simulink model "CobiCalibration"  (R2020b)
settings: Solver=FixedStepDiscrete  StartTime=0.0  StopTime=inf  FixedStep=0.01  RelTol=1e-3  EnableMultiTasking=on
libraries: simulink x9
settings Model: DataDictionary=CobiCalibrationDD.sldd  EnableAccessToBaseWorkspace=off  DataTypeOverride=Off  DataTypeOverrideAppliesTo=Floating-point  MinMaxOverflowLogging=ForceOff  Creator=stj1si  LastModifiedBy=snj7rt
settings DataIOCC: SaveFormat=Array  SaveOutput=off  SignalLogging=off  SaveTime=off  ReturnWorkspaceOutputs=off
settings OptimizationCC: DefaultParameterBehavior=Inlined  DefaultUnderspecifiedDataType=single  InlineInvariantSignals=on  EnhancedBackFolding=on  CachingGlobalReferences=on  ExpressionDepthLimit=2147483647  NoFixptDivByZeroProtection=on  EfficientFloat2IntCast=on  LifeSpan=1  SimCompilerOptimization=on  EfficientTunableParamExpr=on
settings DebuggingCC: SolverPrmCheckMsg=warning  ParameterPrecisionLossMsg=none  AllowSymbolicDim=off  StateNameClashWarn=warning  SFUnexpectedBacktrackingDiag=warning  SFNoUnconditionalDefaultTransitionDiag=warning  SFExecutionAtInitializationDiag=none  ArithmeticOperatorsInVariantConditions=warning
settings HardwareCC: ProdBitPerPointer=32  ProdBitPerSizeT=32  ProdBitPerPtrDiffT=32  ProdLargestAtomicInteger=Long  ProdLargestAtomicFloat=Double  ProdEndianess=BigEndian  ProdWordSize=32  ProdHWDeviceType=Freescale->32-bit PowerPC
settings ModelReferenceCC: ModelReferenceNumInstancesAllowed=Single  PropagateSignalLabelsOutOfModel=off
settings SFSimCC: SimUseLocalCustomCode=off  MATLABDynamicMemAlloc=off  CustomCodeUndefinedFunction=UseInterfaceOnly
settings RTWCC: Description=Embedded Coder  SystemTargetFile=ert.tlc  GenCodeOnly=on  TemplateMakefile=ert_default_tmf  GenerateReport=on  RTWUseLocalCustomCode=off  IncludeHyperlinkInReport=on  LaunchReport=on  GenerateTraceInfo=on  GenerateTraceReport=on  GenerateTraceReportSl=on  GenerateTraceReportSf=on  GenerateTraceReportEml=on
settings CodeAppCC: IgnoreCustomStorageClasses=off  CustomSymbolStrType=$N$R$M  CustomSymbolStrFcnArg=COCA_rt$I$N$M  CustomSymbolStrBlkIO=COCA_rtb_$N$M  StateflowObjectComments=on  InternalIdentifier=Classic
settings ERTTargetCC: TargetLangStandard=C99 (ISO)  MultiwordLength=2048  GenerateSampleERTMain=on  IncludeMdlTerminateFcn=off  CombineSignalStateStructs=on  SuppressErrorStatus=on  SupportNonFinite=off  SupportComplex=off  CastingMode=Standards  InlinedParameterPlacement=NonHierarchical  ERTSrcFileBannerTemplate=ert_code_template_ebike.cgt  ERTCustomFileTemplate=example_file_process.tlc  ERTFilePackagingFormat=Compact  PreserveExternInFcnDecls=off  SuppressUnreachableDefaultCases=off  EnableSignedLeftShifts=off  EnableSignedRightShifts=off  IndentStyle=Allman  EnableUserReplacementTypes=on
settings ConfigComp: CovEnable=on  CovScope=ReferencedModels  CovIncludeTopModel=off  CovMetricSettings=dw  CovHTMLOptions=-sRT=1 -sVT=0 -aTS=1 -bRG=1 -bTC=1 -hTR=0 -nFC=0 -nFD=1 -scm=1 -bcm=1 -xEv=0 -xEM=0  CovSaveCumulativeToWorkspaceVar=on  CovSaveSingleToWorkspaceVar=on  CovModelRefEnable=all  CovSFcnEnable=off

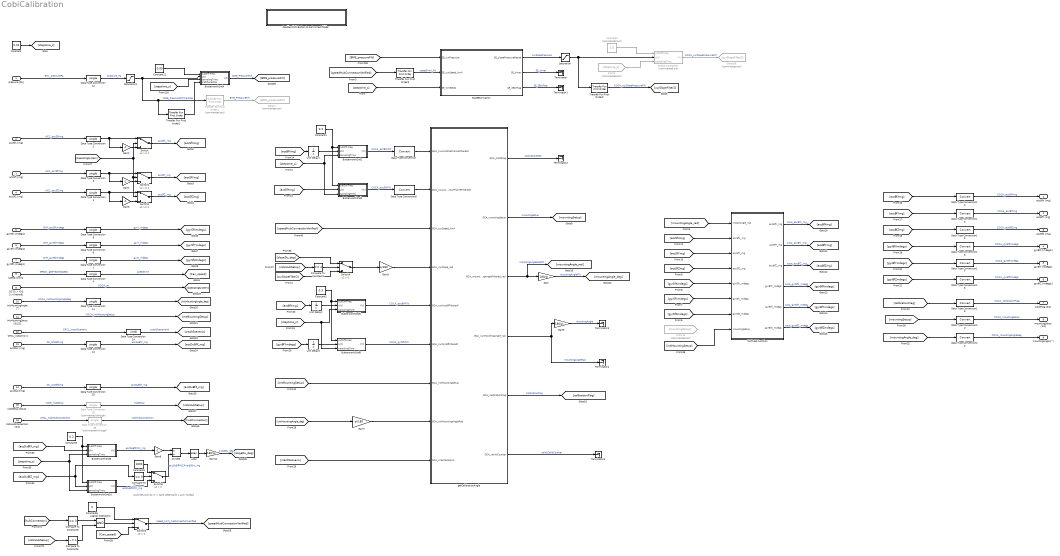
== system CobiCalibration ==
  note: avoid devision by 0 -> take 1000mg for z axis instead
  "pressure [Pa] " : Inport
  accSfX [mg] : Inport  Port=2
  accSfY [mg] : Inport  Port=3
  accSfZ [mg] : Inport  Port=4
  gyrSfX [mdeg/s] : Inport  Port=5
  gyrSfY [mdeg/s] : Inport  Port=6
  gyrSfZ [mdeg/s] : Inport  Port=7
  speed [km/h] : Inport  Port=8
  "OS [1-> iOS, 2->Android]" : Inport  Port=9
  initMountingAngle [°] : Inport  Port=10
  initMountingSetup [0/1/2] : Inport  Port=11
  " CRCL_sceanrio []" : Inport  Port=12
  accDuX [mg] : Inport  Port=13
  accDuZ [mg] : Inport  Port=14
  cobiSetup [0/1/2] : Inport  Port=15
  CobiHubConnection [0/1] : Inport  Port=16
  Atan : Trigonometry  Operator=atan
  Butterworth2nd1 : Subsystem
  Butterworth2nd10 : Subsystem
  Butterworth2nd2 : Subsystem
  Butterworth2nd4 : Subsystem
  Butterworth2nd5 : Subsystem
  Butterworth2nd7 : Subsystem  Commented=on
  Butterworth2nd8 : Subsystem
  Butterworth2nd9 : Subsystem
  Compare To Constant : simulink/Logic and Bit Operations/Compare To Constant  relop===  const=0  OutDataTypeStr=boolean
  Compare To Constant1 : simulink/Logic and Bit Operations/Compare To Constant  relop===  const=2  OutDataTypeStr=boolean
  Compare To Constant6 : simulink/Logic and Bit Operations/Compare To Constant  relop===  const=0  OutDataTypeStr=boolean
  Compare To Constant8 : simulink/Logic and Bit Operations/Compare To Constant  relop=~=  const=1  OutDataTypeStr=boolean
  Constant : Constant  Value=0.01
  Constant1 : Constant  Value=0.3
  Constant11 : Constant  Value=0.05
  Constant2 : Constant  Value=0.3
  Constant3 : Constant  Value=0.2
  Constant4 : Constant  Commented=on  Value=0.5
  Constant5 : Constant  Value=0  OutDataTypeStr=single
  Constant6 : Constant  Value=1000
  Data Type Conversion{,5,10,13,15..19,22..23} (11 alike) : DataTypeConversion  RndMeth=Zero
  Data Type Conversion{1..4,7..9,11..12,24..25} (11 alike) : DataTypeConversion  OutDataTypeStr=single
  Data Type Conversion14 : DataTypeConversion  OutDataTypeStr=uint8
  Data Type Conversion26 : DataTypeConversion  Commented=through  OutDataTypeStr=single
  Data Type Conversion39 : DataTypeConversion  Commented=through  OutDataTypeStr=single
  Divide3 : Product  Inputs=*/
  Double-Click Button to set current folder : Subsystem
      settings: OpenFcn=cd(fileparts(get_param(gcs,'filename')));
      mask Display: disp('\bf\fontsize{16}Double-Click to set current folder      ','texmode','on')
  From1 : From  Commented=on  GotoTag=steptime_s
  From12 : From  Commented=on  GotoTag=mountingSetup
  Gain : Gain  Gain=180/pi
  Gain{1..2,6,8} (4 alike) : Gain  Gain=-1
  Gain12 : Gain  Gain=180/pi
  Gain3 : Gain  Gain=pi/180
  Gain5 : Gain  Gain=180/pi
  Gain7 : Gain  Gain=pi/180
  Goto109 : Goto  Commented=on  GotoTag=curSlopeFilter2
  Goto17 : Goto  Commented=on  GotoTag=BME_pressureFilt
  Logical Operator2 : Logic  AllPortsSameDT=off  OutDataTypeStr=boolean
  MATLAB Function : MATLAB Function  TreatAsAtomicUnit=on
  Saturation : Saturate  UpperLimit=20  LowerLimit=-20
  Saturation1 : Saturate  UpperLimit=120000  LowerLimit=80000
  SlopeEstimation : Stateflow chart  TreatAsAtomicUnit=on
  Switch : Switch  Threshold=2
  Switch1 : Switch  Threshold=2
  Switch2 : Switch  Threshold=2
  Switch3 : Switch  Criteria=u2 > Threshold
  Switch4 : Switch  Criteria=u2 > Threshold
  Switch5 : Switch  Criteria=u2 > Threshold
  Terminator{,1..5} (6 alike) : Terminator
  Transfer Fcn First Order1 : simulink/Discrete/Transfer Fcn First Order  Commented=on  PoleZ=0.995  ICPrevOutput=90000  DoSatur=off
  Transfer Fcn First Order2 : simulink/Discrete/Transfer Fcn First Order  PoleZ=0.95  ICPrevOutput=90000  DoSatur=off
  Transfer Fcn First Order3 : simulink/Discrete/Transfer Fcn First Order  PoleZ=0.995  ICPrevOutput=0  DoSatur=off
  Transfer Fcn First Order9 : simulink/Discrete/Transfer Fcn First Order  PoleZ=0.99  ICPrevOutput=0.0  DoSatur=off
  Unit Delay1 : UnitDelay  SampleTime=-1  HasFrameUpgradeWarning=on
  Unit Delay2 : UnitDelay  SampleTime=-1  HasFrameUpgradeWarning=on
  Unit Delay3 : UnitDelay  SampleTime=-1  HasFrameUpgradeWarning=on
  getCalibrationAngle : Stateflow chart  TreatAsAtomicUnit=on
  accBfX [mg] : Outport  VectorParamsAs1DForOutWhenUnconnected=off
  accBfY [mg] : Outport  Port=2  VectorParamsAs1DForOutWhenUnconnected=off
  accBfZ [mg] : Outport  Port=3  VectorParamsAs1DForOutWhenUnconnected=off
  gyrBfX [mdeg/s] : Outport  Port=4  VectorParamsAs1DForOutWhenUnconnected=off
  gyrBfY [mdeg/s] : Outport  Port=5  VectorParamsAs1DForOutWhenUnconnected=off
  gyrBfZ [mdeg/s] : Outport  Port=6  VectorParamsAs1DForOutWhenUnconnected=off
  calibFlag [0/1] : Outport  Port=7  VectorParamsAs1DForOutWhenUnconnected=off
  mountingSetup [1/2] : Outport  Port=8  VectorParamsAs1DForOutWhenUnconnected=off
  mountingAngle [°] : Outport  Port=9  VectorParamsAs1DForOutWhenUnconnected=off
  wires:
  accSfY [mg]/1 -> Data Type Conversion3/1  "ACC_accSfYmg"
  accSfX [mg]/1 -> Data Type Conversion2/1  "ACC_accSfXmg"
  "pressure [Pa] "/1 -> Data Type Conversion12/1  "ENV_pressurePa"
  accSfZ [mg]/1 -> Data Type Conversion1/1  "ACC_accSfZmg"
  gyrSfX [mdeg/s]/1 -> Data Type Conversion8/1  "GYR_gyrSfXmdegs"
  gyrSfY [mdeg/s]/1 -> Data Type Conversion9/1  "GYR_gyrSfYmdegs"
  gyrSfZ [mdeg/s]/1 -> Data Type Conversion7/1  "GYR_gyrSfZmdegs"
  Data Type Conversion10/1 -> accBfX [mg]/1  "COCA_accBfXmg"
  Data Type Conversion13/1 -> accBfY [mg]/1  "COCA_accBfYmg"
  Data Type Conversion15/1 -> accBfZ [mg]/1  "COCA_accBfZmg"
  Data Type Conversion16/1 -> gyrBfX [mdeg/s]/1  "COCA_gyrBfXmdegs"
  Data Type Conversion17/1 -> gyrBfY [mdeg/s]/1  "COCA_gyrBfYmdegs"
  Data Type Conversion18/1 -> gyrBfZ [mdeg/s]/1  "COCA_gyrBfZmdegs"
  Data Type Conversion12/1 -> Saturation1/1  "pressure_Pa"
  Data Type Conversion2/1 -> Switch/1, Gain2/1
  Data Type Conversion1/1 -> Gain6/1, Switch2/1
  Data Type Conversion8/1 -> [gyrSfXmdegs]  "gyrX_mdegs"
  Data Type Conversion9/1 -> [gyrSfYmdegs]  "gyrY_mdegs"
  Data Type Conversion7/1 -> [gyrSfZmdegs]  "gyrZ_mdegs"
  Constant11/1 -> Butterworth2nd4/1(cutOff-Freq)
  [steptime_s] -> Butterworth2nd4/3(samplingTime)
  Butterworth2nd4/1(Y(t)) -> [BME_pressureFilt]  "BME_PressureFilt"
  Constant/1 -> [steptime_s]
  Butterworth2nd7/1(Y(t)) -> Goto109/1  "COCA_curSlopePressureFilt"
  [steptime_s] -> SlopeEstimation/3(SE_timeStep)
  From1/1 -> Butterworth2nd7/3(samplingTime)
  [BME_pressureFilt] -> SlopeEstimation/1(SE_curPressure)
  SlopeEstimation/1(SE_slopePressureBased) -> Saturation/1  "curSlopePressure"
  Constant4/1 -> Butterworth2nd7/1(cutOff-Freq)
  [speedHubConnectionVerified] -> Transfer Fcn First Order3/1
  speed [km/h]/1 -> Data Type Conversion4/1  "SPECO_getPresentSpeed"
  Constant1/1 -> Butterworth2nd2/1(cutOff-Freq), Butterworth2nd1/1(cutOff-Freq)
  [steptime_s] -> Butterworth2nd1/3(samplingTime), Butterworth2nd2/3(samplingTime)
  Butterworth2nd1/1(Y(t)) -> Data Type Conversion/1  "COCA_accBfXFilt"
  Butterworth2nd2/1(Y(t)) -> Data Type Conversion5/1  "COCA_accSfXFilt"
  [speedHubConnectionVerified] -> getCalibrationAngle/3(GCA_curSpeed_kmh)
  getCalibrationAngle/2(GCA_mountingSetup) -> [mountingSetup]  "mountingSetup"
  getCalibrationAngle/4(GCA_curMountingAngle_rad) -> Terminator4/1, Gain5/1  "mountingAngleRad"
  [mountingAngle_rad] -> MATLAB Function/1(installAngle_rad)
  [accSfXmg] -> MATLAB Function/2(accSfX_mg)
  [accSfYmg] -> MATLAB Function/3(accSfY_mg)
  [accSfZmg] -> MATLAB Function/4(accSfZ_mg)
  [gyrSfXmdegs] -> MATLAB Function/5(gyrSfX_mdegs)
  [gyrSfYmdegs] -> MATLAB Function/6(gyrSfY_mdegs)
  [gyrSfZmdegs] -> MATLAB Function/7(gyrSfZ_mdegs)
  [accSfXmg] -> Butterworth2nd2/2(U(t))
  MATLAB Function/5(gyrBfY_mdegs) -> [gyrBfYmdegs]  "coca_gyrBfY_mdegs"
  MATLAB Function/6(gyrBfZ_mdegs) -> [gyrBfZmdegs]  "coca_gyrBfZ_mdegs"
  MATLAB Function/4(gyrBfX_mdegs) -> [gyrBfXmdegs]  "coca_gyrBfX_mdegs"
  MATLAB Function/3(accBfZ_mg) -> [accBfZmg]  "coca_accBfZ_mg"
  MATLAB Function/2(accBfY_mg) -> [accBfYmg]  "coca_accBfY_mg"
  MATLAB Function/1(accBfX_mg) -> [accBfXmg]  "coca_accBfX_mg"
  [accBfXmg] -> Unit Delay1/1
  getCalibrationAngle/3(GCA_mountingAngleFitlered_rad) -> [mountingAngle_rad], Gain/1  "mountingAngleRadFilt"
  getCalibrationAngle/1(GCA_calibFlag) -> Terminator2/1  "calibrationStep"
  [accBfXmg] -> Data Type Conversion10/1
  [accBfYmg] -> Data Type Conversion13/1
  [accBfZmg] -> Data Type Conversion15/1
  [gyrBfXmdegs] -> Data Type Conversion16/1
  [gyrBfYmdegs] -> Data Type Conversion17/1
  [gyrBfZmdegs] -> Data Type Conversion18/1
  Unit Delay1/1 -> Butterworth2nd1/2(U(t))
  Data Type Conversion/1 -> getCalibrationAngle/1(GCA_curAccBikeFrameFilteredX)
  Data Type Conversion5/1 -> getCalibrationAngle/2(GCA_curAccSensorFrameFilteredX)
  [curSlopeFilter2] -> Switch4/3
  Transfer Fcn First Order9/1 -> [curSlopeFilter2]  "COCA_curSlopePressureFilt"
  Transfer Fcn First Order1/1 -> Goto17/1  "BME_PressureFilt"
  Transfer Fcn First Order2/1 -> Butterworth2nd4/4(prefilteredVal)  "BME_PressureFiltTransFer"
  Gain3/1 -> getCalibrationAngle/4(GCA_curSlope_rad)
  getCalibrationAngle/5(GCA_calibrationFlag) -> [calibrationFlag]  "calibrationFlag"
  Data Type Conversion19/1 -> calibFlag [0/1]/1  "COCA_calibrationFlag"
  [calibrationFlag] -> Data Type Conversion19/1
  Butterworth2nd5/1(Y(t)) -> getCalibrationAngle/5(GCA_curAccBfFilteredY)  "COCA_accBfYFilt"
  [accBfYmg] -> Unit Delay2/1
  Unit Delay2/1 -> Butterworth2nd5/2(U(t))
  [steptime_s] -> Butterworth2nd8/3(samplingTime), Butterworth2nd5/3(samplingTime)
  Saturation1/1 -> Butterworth2nd4/2(U(t)), Transfer Fcn First Order2/1, Transfer Fcn First Order1/1
  Data Type Conversion4/1 -> [Can_speed]  "speedKmh"
  Gain/1 -> [mountingAngle_deg]  "mountingAngleFilt"
  Gain5/1 -> Terminator3/1  "mountingAngle"
  getCalibrationAngle/6(GCA_reinitCounter) -> Terminator5/1  "reinitCalibCounter"
  Saturation/1 -> Transfer Fcn First Order9/1, Butterworth2nd7/2(U(t))
  Transfer Fcn First Order3/1 -> SlopeEstimation/2(SE_curSpeed_kmh)  "speedKmh_filt"
  SlopeEstimation/2(SE_timer) -> Terminator/1  "SE_timer"
  SlopeEstimation/3(SE_2EstFlag) -> Terminator1/1  "SE_2EstFalg"
  [gyrBfYmdegs] -> Unit Delay3/1
  Constant2/1 -> Butterworth2nd8/1(cutOff-Freq), Butterworth2nd5/1(cutOff-Freq)
  Butterworth2nd8/1(Y(t)) -> getCalibrationAngle/6(GCA_curGyrBfFilteredY)  "COCA_gyrBfYFilt"
  Unit Delay3/1 -> Butterworth2nd8/2(U(t))
  "OS [1-> iOS, 2->Android]"/1 -> [OperatingSystem]  "COCA_os"
  Switch/1 -> [accSfXmg]  "accSfX_mg"
  Gain2/1 -> Switch/3
  Gain1/1 -> Switch1/3
  [OperatingSystem] -> Switch2/2, Switch1/2, Switch/2
  Switch1/1 -> [accSfYmg]  "accSfY_mg"
  Data Type Conversion3/1 -> Gain1/1, Switch1/1
  Switch2/1 -> [accSfZmg]  "accSfZ_mg"
  Gain6/1 -> Switch2/3
  initMountingAngle [°]/1 -> Data Type Conversion11/1  "COCA_initMountingAngleDeg"
  initMountingSetup [0/1/2]/1 -> [initMountingSetup]  "COCA_initMountingSetup"
  Data Type Conversion22/1 -> mountingSetup [1/2]/1  "COCA_mountingSetup"
  [mountingSetup] -> Data Type Conversion22/1
  Data Type Conversion23/1 -> mountingAngle [°]/1  "COCA_mountingAngleDeg"
  [mountingAngle_deg] -> Data Type Conversion23/1
  [initMountingSetup] -> getCalibrationAngle/7(GCA_initMountingSetup)
  [initMountingAngle_deg] -> Gain7/1
  Gain7/1 -> getCalibrationAngle/8(GCA_initMountingAngleRad)
  " CRCL_sceanrio []"/1 -> Data Type Conversion14/1  "CRCL_crashScenario"
  [crashScenario] -> getCalibrationAngle/9(GCA_crashScenario)
  accDuX [mg]/1 -> Data Type Conversion24/1  "DU_accBfXmg"
  accDuZ [mg]/1 -> Data Type Conversion25/1  "DU_accBfZmg"
  Data Type Conversion24/1 -> [accDuBfX_mg]  "accDuBfX_mg"
  Data Type Conversion25/1 -> [accDuBfZ_mg]  "accDuBfZ_mg"
  [steptime_s] -> Butterworth2nd10/3(samplingTime), Butterworth2nd9/3(samplingTime)
  Constant3/1 -> Butterworth2nd10/1(cutOff-Freq), Butterworth2nd9/1(cutOff-Freq)
  [accDuBfX_mg] -> Butterworth2nd9/2(U(t))
  [accDuBfZ_mg] -> Compare To Constant/1, Butterworth2nd10/2(U(t))
  Butterworth2nd10/1(Y(t)) -> Switch5/3  "accDuBfFiltZ_mg"
  Butterworth2nd9/1(Y(t)) -> Gain8/1  "accDuBfFiltX_mg"
  Divide3/1 -> Atan/1
  Atan/1 -> Gain12/1
  Gain12/1 -> [slopeDu_deg]  "slopeDu_deg"
  cobiSetup [0/1/2]/1 -> Data Type Conversion26/1  "COBI_hubSetup"
  Data Type Conversion26/1 -> [cobiHubSetup]  "hubSetup"
  Gain8/1 -> Divide3/1
  Switch4/1 -> Gain3/1
  Compare To Constant1/1 -> Switch4/2
  [slopeDu_deg] -> Switch4/1
  [cobiHubSetup] -> Compare To Constant1/1
  [initMountingSetup] -> MATLAB Function/8(mountingSetup)
  Data Type Conversion11/1 -> [initMountingAngle_deg]
  Data Type Conversion39/1 -> [hubConnection]  "cobiHubConnection"
  CobiHubConnection [0/1]/1 -> Data Type Conversion39/1  "CRCL_CobiHubConnection"
  Constant5/1 -> Switch3/1
  Compare To Constant6/1 -> Logical Operator2/1
  [cobiHubSetup] -> Compare To Constant8/1
  Logical Operator2/1 -> Switch3/2
  [hubConnection] -> Compare To Constant6/1
  [Can_speed] -> Switch3/3
  Compare To Constant8/1 -> Logical Operator2/2
  Switch3/1 -> [speedHubConnectionVerified]  "speed_kmh_hubConnectionVerified"
  Compare To Constant/1 -> Switch5/2
  Switch5/1 -> Divide3/2  "accDuBfFiltZAvoid0Div_mg"
  Constant6/1 -> Switch5/1
  Data Type Conversion14/1 -> [crashScenario]  "crashScenarioInt"

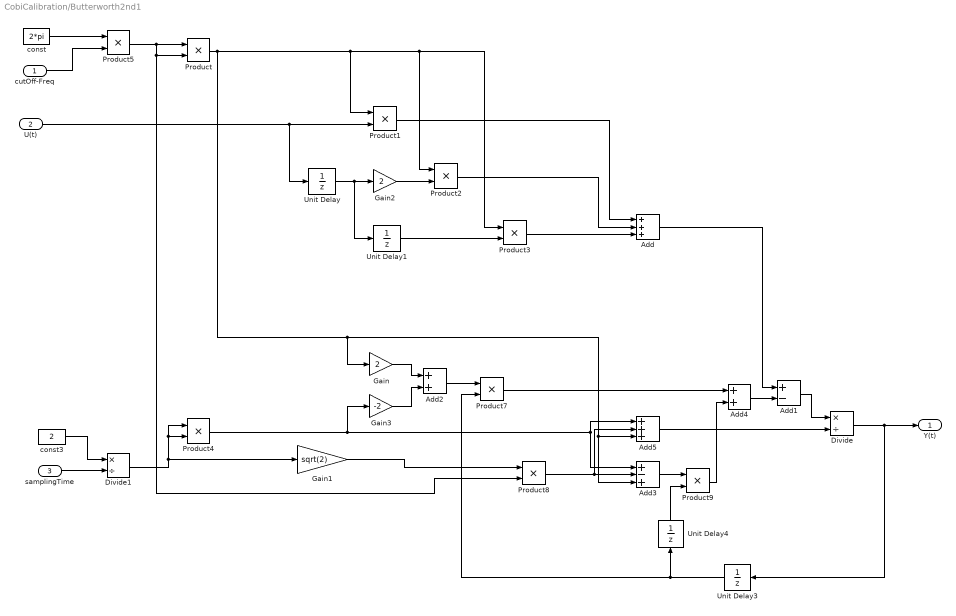
== system CobiCalibration/Butterworth2nd1 ==
  cutOff-Freq : Inport
  U(t) : Inport  Port=2
  samplingTime : Inport  Port=3
  Add : Sum  Inputs=+++
  Add1 : Sum  Inputs=+-
  Add2 : Sum
  Add3 : Sum  Inputs=+-+
  Add4 : Sum
  Add5 : Sum  Inputs=+++
  Divide : Product  Inputs=*/
  Divide1 : Product  Inputs=*/
  Gain : Gain  Gain=2
  Gain1 : Gain  Gain=sqrt(2)
  Gain2 : Gain  Gain=2
  Gain3 : Gain  Gain=-2
  Product{,1..5,7..9} (9 alike) : Product  RndMeth=Zero
  Unit Delay{,1,3..4} (4 alike) : UnitDelay  SampleTime=-1  HasFrameUpgradeWarning=on
  const : Constant  Value=2*pi
  const3 : Constant  Value=2
  Y(t) : Outport  VectorParamsAs1DForOutWhenUnconnected=off
  wires:
  U(t)/1 -> Product1/2, Unit Delay/1
  Product/1 -> Product1/1, Product3/1, Product2/1, Gain/1, Add3/3, Add5/3
  Unit Delay/1 -> Unit Delay1/1, Gain2/1
  Unit Delay1/1 -> Product3/2
  Product1/1 -> Add/1
  Product2/1 -> Add/2
  Product3/1 -> Add/3
  Add/1 -> Add1/1
  Divide/1 -> Unit Delay3/1, Y(t)/1
  Product4/1 -> Add3/1, Add5/1, Gain3/1
  Gain/1 -> Add2/1
  Unit Delay3/1 -> Product7/2, Unit Delay4/1
  Add2/1 -> Product7/1
  Gain1/1 -> Product8/1
  Product8/1 -> Add3/2, Add5/2
  Unit Delay4/1 -> Product9/2
  Add3/1 -> Product9/1
  Product9/1 -> Add4/2
  Product7/1 -> Add4/1
  Add4/1 -> Add1/2
  Add1/1 -> Divide/1
  Add5/1 -> Divide/2
  Gain2/1 -> Product2/2
  Gain3/1 -> Add2/2
  Product5/1 -> Product/1, Product/2, Product8/2
  const/1 -> Product5/1
  cutOff-Freq/1 -> Product5/2
  const3/1 -> Divide1/1
  samplingTime/1 -> Divide1/2
  Divide1/1 -> Gain1/1, Product4/2, Product4/1

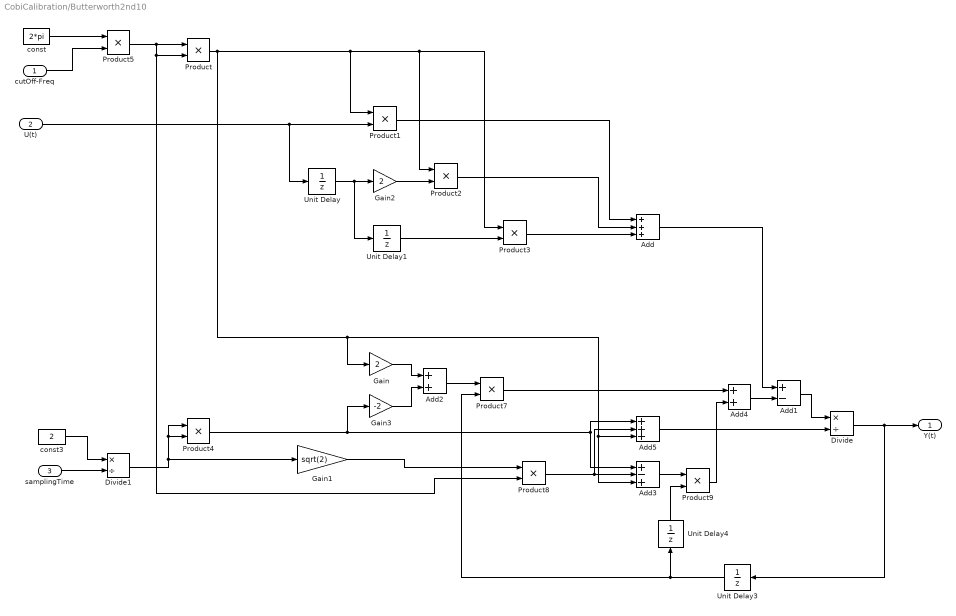
== system CobiCalibration/Butterworth2nd10 ==
  cutOff-Freq : Inport
  U(t) : Inport  Port=2
  samplingTime : Inport  Port=3
  Add : Sum  Inputs=+++
  Add1 : Sum  Inputs=+-
  Add2 : Sum
  Add3 : Sum  Inputs=+-+
  Add4 : Sum
  Add5 : Sum  Inputs=+++
  Divide : Product  Inputs=*/
  Divide1 : Product  Inputs=*/
  Gain : Gain  Gain=2
  Gain1 : Gain  Gain=sqrt(2)
  Gain2 : Gain  Gain=2
  Gain3 : Gain  Gain=-2
  Product{,1..5,7..9} (9 alike) : Product  RndMeth=Zero
  Unit Delay : UnitDelay  SampleTime=-1  HasFrameUpgradeWarning=on
  Unit Delay1 : UnitDelay  SampleTime=-1  HasFrameUpgradeWarning=on
  Unit Delay3 : UnitDelay  InitialCondition=1000  SampleTime=-1  HasFrameUpgradeWarning=on
  Unit Delay4 : UnitDelay  InitialCondition=1000  SampleTime=-1  HasFrameUpgradeWarning=on
  const : Constant  Value=2*pi
  const3 : Constant  Value=2
  Y(t) : Outport  VectorParamsAs1DForOutWhenUnconnected=off
  wires:
  Divide1/1 -> Product4/1, Product4/2, Gain1/1
  samplingTime/1 -> Divide1/2
  const3/1 -> Divide1/1
  cutOff-Freq/1 -> Product5/2
  const/1 -> Product5/1
  Product5/1 -> Product8/2, Product/2, Product/1
  Gain3/1 -> Add2/2
  Gain2/1 -> Product2/2
  Add5/1 -> Divide/2
  Add1/1 -> Divide/1
  Add4/1 -> Add1/2
  Product7/1 -> Add4/1
  Product9/1 -> Add4/2
  Add3/1 -> Product9/1
  Unit Delay4/1 -> Product9/2
  Product8/1 -> Add5/2, Add3/2
  Gain1/1 -> Product8/1
  Add2/1 -> Product7/1
  Unit Delay3/1 -> Unit Delay4/1, Product7/2
  Gain/1 -> Add2/1
  Product4/1 -> Gain3/1, Add5/1, Add3/1
  Divide/1 -> Y(t)/1, Unit Delay3/1
  Add/1 -> Add1/1
  Product3/1 -> Add/3
  Product2/1 -> Add/2
  Product1/1 -> Add/1
  Unit Delay1/1 -> Product3/2
  Unit Delay/1 -> Gain2/1, Unit Delay1/1
  Product/1 -> Add5/3, Add3/3, Gain/1, Product2/1, Product3/1, Product1/1
  U(t)/1 -> Unit Delay/1, Product1/2

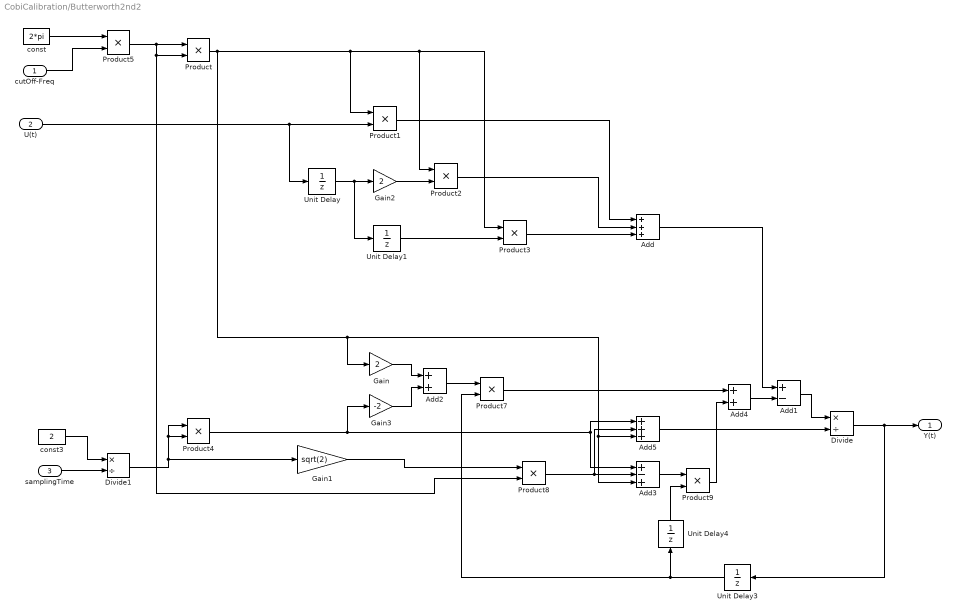
== system CobiCalibration/Butterworth2nd2 ==
  cutOff-Freq : Inport
  U(t) : Inport  Port=2
  samplingTime : Inport  Port=3
  Add : Sum  Inputs=+++
  Add1 : Sum  Inputs=+-
  Add2 : Sum
  Add3 : Sum  Inputs=+-+
  Add4 : Sum
  Add5 : Sum  Inputs=+++
  Divide : Product  Inputs=*/
  Divide1 : Product  Inputs=*/
  Gain : Gain  Gain=2
  Gain1 : Gain  Gain=sqrt(2)
  Gain2 : Gain  Gain=2
  Gain3 : Gain  Gain=-2
  Product{,1..5,7..9} (9 alike) : Product  RndMeth=Zero
  Unit Delay{,1,3..4} (4 alike) : UnitDelay  SampleTime=-1  HasFrameUpgradeWarning=on
  const : Constant  Value=2*pi
  const3 : Constant  Value=2
  Y(t) : Outport  VectorParamsAs1DForOutWhenUnconnected=off
  wires:
  Divide1/1 -> Product4/1, Product4/2, Gain1/1
  samplingTime/1 -> Divide1/2
  const3/1 -> Divide1/1
  cutOff-Freq/1 -> Product5/2
  const/1 -> Product5/1
  Product5/1 -> Product8/2, Product/2, Product/1
  Gain3/1 -> Add2/2
  Gain2/1 -> Product2/2
  Add5/1 -> Divide/2
  Add1/1 -> Divide/1
  Add4/1 -> Add1/2
  Product7/1 -> Add4/1
  Product9/1 -> Add4/2
  Add3/1 -> Product9/1
  Unit Delay4/1 -> Product9/2
  Product8/1 -> Add5/2, Add3/2
  Gain1/1 -> Product8/1
  Add2/1 -> Product7/1
  Unit Delay3/1 -> Unit Delay4/1, Product7/2
  Gain/1 -> Add2/1
  Product4/1 -> Gain3/1, Add5/1, Add3/1
  Divide/1 -> Y(t)/1, Unit Delay3/1
  Add/1 -> Add1/1
  Product3/1 -> Add/3
  Product2/1 -> Add/2
  Product1/1 -> Add/1
  Unit Delay1/1 -> Product3/2
  Unit Delay/1 -> Gain2/1, Unit Delay1/1
  Product/1 -> Add5/3, Add3/3, Gain/1, Product2/1, Product3/1, Product1/1
  U(t)/1 -> Unit Delay/1, Product1/2

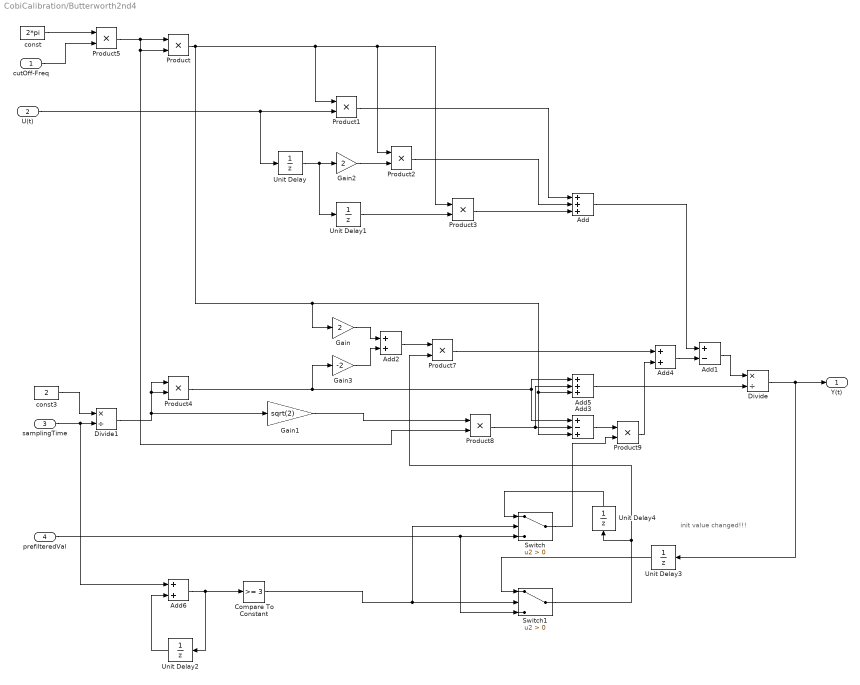
== system CobiCalibration/Butterworth2nd4 ==
  note: init value changed!!!
  cutOff-Freq : Inport
  U(t) : Inport  Port=2
  samplingTime : Inport  Port=3
  prefilteredVal : Inport  Port=4
  Add : Sum  Inputs=+++
  Add1 : Sum  Inputs=+-
  Add2 : Sum
  Add3 : Sum  Inputs=+-+
  Add4 : Sum
  Add5 : Sum  Inputs=+++
  Add6 : Sum
  Compare To Constant : simulink/Logic and Bit Operations/Compare To Constant  relop=>=  const=3  OutDataTypeStr=boolean
  Divide : Product  Inputs=*/
  Divide1 : Product  Inputs=*/
  Gain : Gain  Gain=2
  Gain1 : Gain  Gain=sqrt(2)
  Gain2 : Gain  Gain=2
  Gain3 : Gain  Gain=-2
  Product{,1..5,7..9} (9 alike) : Product  RndMeth=Zero
  Switch : Switch  Criteria=u2 > Threshold
  Switch1 : Switch  Criteria=u2 > Threshold
  Unit Delay{,1..4} (5 alike) : UnitDelay  SampleTime=-1  HasFrameUpgradeWarning=on
  const : Constant  Value=2*pi
  const3 : Constant  Value=2
  Y(t) : Outport  VectorParamsAs1DForOutWhenUnconnected=off
  wires:
  Divide1/1 -> Product4/1, Product4/2, Gain1/1
  samplingTime/1 -> Add6/1, Divide1/2
  const3/1 -> Divide1/1
  cutOff-Freq/1 -> Product5/2
  const/1 -> Product5/1
  Product5/1 -> Product8/2, Product/2, Product/1
  Gain3/1 -> Add2/2
  Gain2/1 -> Product2/2
  Add5/1 -> Divide/2
  Add1/1 -> Divide/1
  Add4/1 -> Add1/2
  Product7/1 -> Add4/1
  Product9/1 -> Add4/2
  Add3/1 -> Product9/1
  Unit Delay4/1 -> Switch/1
  Product8/1 -> Add5/2, Add3/2
  Gain1/1 -> Product8/1
  Add2/1 -> Product7/1
  Gain/1 -> Add2/1
  Product4/1 -> Gain3/1, Add5/1, Add3/1
  Divide/1 -> Y(t)/1, Unit Delay3/1
  Add/1 -> Add1/1
  Product3/1 -> Add/3
  Product2/1 -> Add/2
  Product1/1 -> Add/1
  Unit Delay1/1 -> Product3/2
  Unit Delay/1 -> Gain2/1, Unit Delay1/1
  Product/1 -> Add5/3, Add3/3, Gain/1, Product2/1, Product3/1, Product1/1
  U(t)/1 -> Unit Delay/1, Product1/2
  prefilteredVal/1 -> Switch1/3, Switch/3
  Switch/1 -> Product9/2
  Unit Delay3/1 -> Switch1/1
  Switch1/1 -> Unit Delay4/1, Product7/2
  Add6/1 -> Compare To Constant/1, Unit Delay2/1
  Unit Delay2/1 -> Add6/2
  Compare To Constant/1 -> Switch/2, Switch1/2

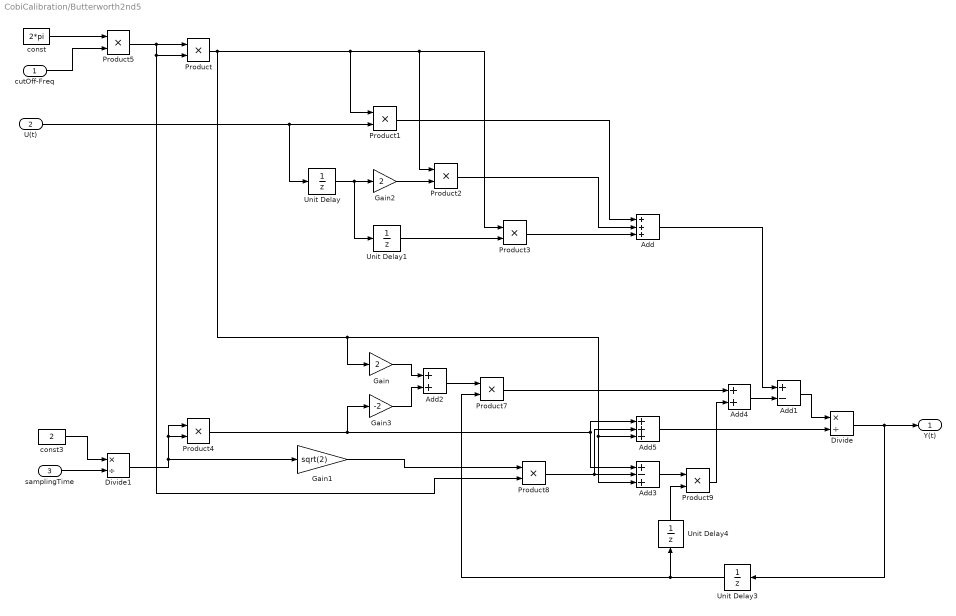
== system CobiCalibration/Butterworth2nd5 ==
  cutOff-Freq : Inport
  U(t) : Inport  Port=2
  samplingTime : Inport  Port=3
  Add : Sum  Inputs=+++
  Add1 : Sum  Inputs=+-
  Add2 : Sum
  Add3 : Sum  Inputs=+-+
  Add4 : Sum
  Add5 : Sum  Inputs=+++
  Divide : Product  Inputs=*/
  Divide1 : Product  Inputs=*/
  Gain : Gain  Gain=2
  Gain1 : Gain  Gain=sqrt(2)
  Gain2 : Gain  Gain=2
  Gain3 : Gain  Gain=-2
  Product{,1..5,7..9} (9 alike) : Product  RndMeth=Zero
  Unit Delay{,1,3..4} (4 alike) : UnitDelay  SampleTime=-1  HasFrameUpgradeWarning=on
  const : Constant  Value=2*pi
  const3 : Constant  Value=2
  Y(t) : Outport  VectorParamsAs1DForOutWhenUnconnected=off
  wires:
  Divide1/1 -> Product4/1, Product4/2, Gain1/1
  samplingTime/1 -> Divide1/2
  const3/1 -> Divide1/1
  cutOff-Freq/1 -> Product5/2
  const/1 -> Product5/1
  Product5/1 -> Product8/2, Product/2, Product/1
  Gain3/1 -> Add2/2
  Gain2/1 -> Product2/2
  Add5/1 -> Divide/2
  Add1/1 -> Divide/1
  Add4/1 -> Add1/2
  Product7/1 -> Add4/1
  Product9/1 -> Add4/2
  Add3/1 -> Product9/1
  Unit Delay4/1 -> Product9/2
  Product8/1 -> Add5/2, Add3/2
  Gain1/1 -> Product8/1
  Add2/1 -> Product7/1
  Unit Delay3/1 -> Unit Delay4/1, Product7/2
  Gain/1 -> Add2/1
  Product4/1 -> Gain3/1, Add5/1, Add3/1
  Divide/1 -> Y(t)/1, Unit Delay3/1
  Add/1 -> Add1/1
  Product3/1 -> Add/3
  Product2/1 -> Add/2
  Product1/1 -> Add/1
  Unit Delay1/1 -> Product3/2
  Unit Delay/1 -> Gain2/1, Unit Delay1/1
  Product/1 -> Add5/3, Add3/3, Gain/1, Product2/1, Product3/1, Product1/1
  U(t)/1 -> Unit Delay/1, Product1/2

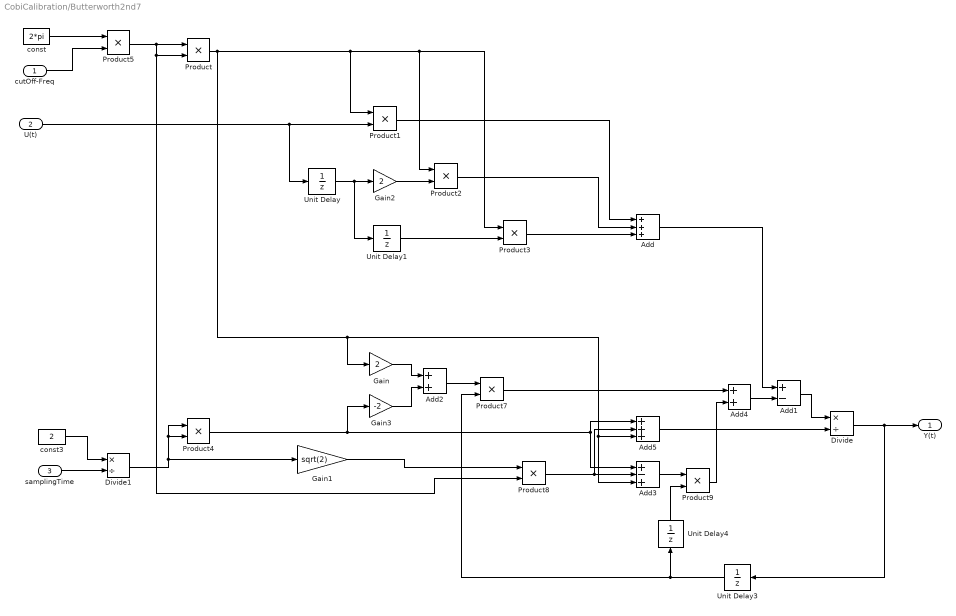
== system CobiCalibration/Butterworth2nd7 ==
  cutOff-Freq : Inport
  U(t) : Inport  Port=2
  samplingTime : Inport  Port=3
  Add : Sum  Inputs=+++
  Add1 : Sum  Inputs=+-
  Add2 : Sum
  Add3 : Sum  Inputs=+-+
  Add4 : Sum
  Add5 : Sum  Inputs=+++
  Divide : Product  Inputs=*/
  Divide1 : Product  Inputs=*/
  Gain : Gain  Gain=2
  Gain1 : Gain  Gain=sqrt(2)
  Gain2 : Gain  Gain=2
  Gain3 : Gain  Gain=-2
  Product{,1..5,7..9} (9 alike) : Product  RndMeth=Zero
  Unit Delay{,1,3..4} (4 alike) : UnitDelay  SampleTime=-1  HasFrameUpgradeWarning=on
  const : Constant  Value=2*pi
  const3 : Constant  Value=2
  Y(t) : Outport  VectorParamsAs1DForOutWhenUnconnected=off
  wires:
  U(t)/1 -> Product1/2, Unit Delay/1
  Product/1 -> Product1/1, Product3/1, Product2/1, Gain/1, Add3/3, Add5/3
  Unit Delay/1 -> Unit Delay1/1, Gain2/1
  Unit Delay1/1 -> Product3/2
  Product1/1 -> Add/1
  Product2/1 -> Add/2
  Product3/1 -> Add/3
  Add/1 -> Add1/1
  Divide/1 -> Unit Delay3/1, Y(t)/1
  Product4/1 -> Add3/1, Add5/1, Gain3/1
  Gain/1 -> Add2/1
  Unit Delay3/1 -> Product7/2, Unit Delay4/1
  Add2/1 -> Product7/1
  Gain1/1 -> Product8/1
  Product8/1 -> Add3/2, Add5/2
  Unit Delay4/1 -> Product9/2
  Add3/1 -> Product9/1
  Product9/1 -> Add4/2
  Product7/1 -> Add4/1
  Add4/1 -> Add1/2
  Add1/1 -> Divide/1
  Add5/1 -> Divide/2
  Gain2/1 -> Product2/2
  Gain3/1 -> Add2/2
  Product5/1 -> Product/1, Product/2, Product8/2
  const/1 -> Product5/1
  cutOff-Freq/1 -> Product5/2
  const3/1 -> Divide1/1
  samplingTime/1 -> Divide1/2
  Divide1/1 -> Gain1/1, Product4/2, Product4/1

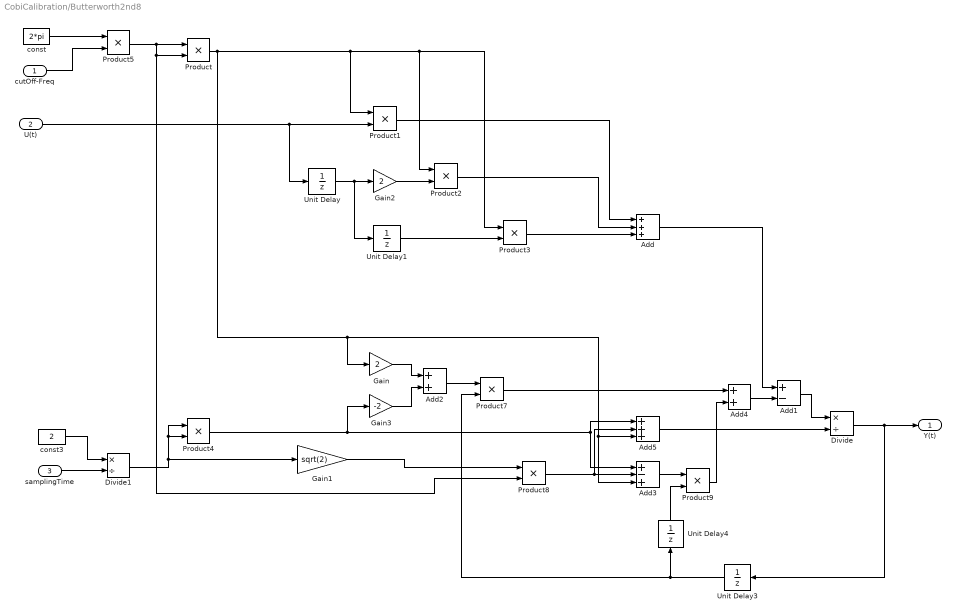
== system CobiCalibration/Butterworth2nd8 ==
  cutOff-Freq : Inport
  U(t) : Inport  Port=2
  samplingTime : Inport  Port=3
  Add : Sum  Inputs=+++
  Add1 : Sum  Inputs=+-
  Add2 : Sum
  Add3 : Sum  Inputs=+-+
  Add4 : Sum
  Add5 : Sum  Inputs=+++
  Divide : Product  Inputs=*/
  Divide1 : Product  Inputs=*/
  Gain : Gain  Gain=2
  Gain1 : Gain  Gain=sqrt(2)
  Gain2 : Gain  Gain=2
  Gain3 : Gain  Gain=-2
  Product{,1..5,7..9} (9 alike) : Product  RndMeth=Zero
  Unit Delay{,1,3..4} (4 alike) : UnitDelay  SampleTime=-1  HasFrameUpgradeWarning=on
  const : Constant  Value=2*pi
  const3 : Constant  Value=2
  Y(t) : Outport  VectorParamsAs1DForOutWhenUnconnected=off
  wires:
  Divide1/1 -> Product4/1, Product4/2, Gain1/1
  samplingTime/1 -> Divide1/2
  const3/1 -> Divide1/1
  cutOff-Freq/1 -> Product5/2
  const/1 -> Product5/1
  Product5/1 -> Product8/2, Product/2, Product/1
  Gain3/1 -> Add2/2
  Gain2/1 -> Product2/2
  Add5/1 -> Divide/2
  Add1/1 -> Divide/1
  Add4/1 -> Add1/2
  Product7/1 -> Add4/1
  Product9/1 -> Add4/2
  Add3/1 -> Product9/1
  Unit Delay4/1 -> Product9/2
  Product8/1 -> Add5/2, Add3/2
  Gain1/1 -> Product8/1
  Add2/1 -> Product7/1
  Unit Delay3/1 -> Unit Delay4/1, Product7/2
  Gain/1 -> Add2/1
  Product4/1 -> Gain3/1, Add5/1, Add3/1
  Divide/1 -> Y(t)/1, Unit Delay3/1
  Add/1 -> Add1/1
  Product3/1 -> Add/3
  Product2/1 -> Add/2
  Product1/1 -> Add/1
  Unit Delay1/1 -> Product3/2
  Unit Delay/1 -> Gain2/1, Unit Delay1/1
  Product/1 -> Add5/3, Add3/3, Gain/1, Product2/1, Product3/1, Product1/1
  U(t)/1 -> Unit Delay/1, Product1/2

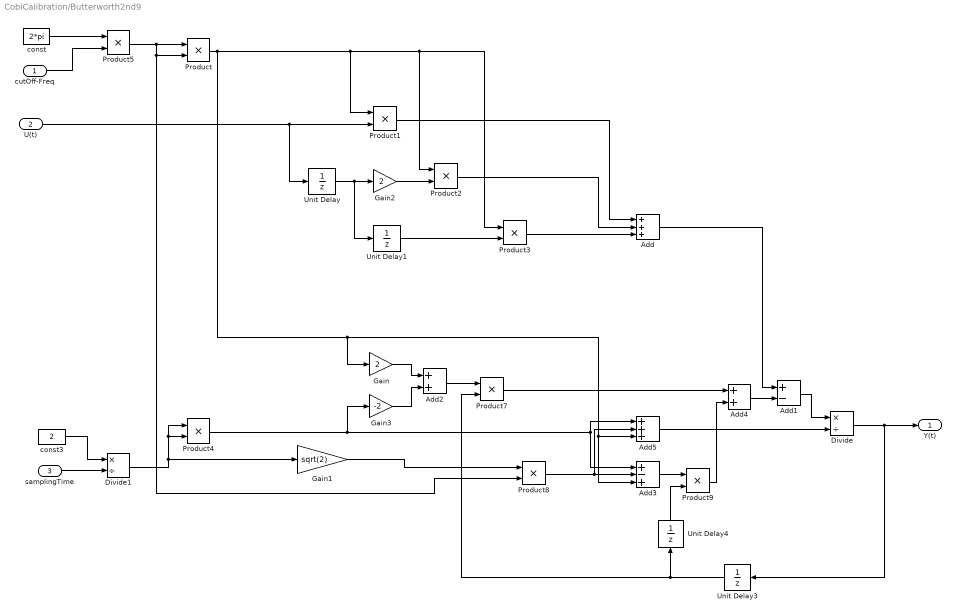
== system CobiCalibration/Butterworth2nd9 ==
  cutOff-Freq : Inport
  U(t) : Inport  Port=2
  samplingTime : Inport  Port=3
  Add : Sum  Inputs=+++
  Add1 : Sum  Inputs=+-
  Add2 : Sum
  Add3 : Sum  Inputs=+-+
  Add4 : Sum
  Add5 : Sum  Inputs=+++
  Divide : Product  Inputs=*/
  Divide1 : Product  Inputs=*/
  Gain : Gain  Gain=2
  Gain1 : Gain  Gain=sqrt(2)
  Gain2 : Gain  Gain=2
  Gain3 : Gain  Gain=-2
  Product{,1..5,7..9} (9 alike) : Product  RndMeth=Zero
  Unit Delay{,1,3..4} (4 alike) : UnitDelay  SampleTime=-1  HasFrameUpgradeWarning=on
  const : Constant  Value=2*pi
  const3 : Constant  Value=2
  Y(t) : Outport  VectorParamsAs1DForOutWhenUnconnected=off
  wires:
  U(t)/1 -> Product1/2, Unit Delay/1
  Product/1 -> Product1/1, Product3/1, Product2/1, Gain/1, Add3/3, Add5/3
  Unit Delay/1 -> Unit Delay1/1, Gain2/1
  Unit Delay1/1 -> Product3/2
  Product1/1 -> Add/1
  Product2/1 -> Add/2
  Product3/1 -> Add/3
  Add/1 -> Add1/1
  Divide/1 -> Unit Delay3/1, Y(t)/1
  Product4/1 -> Add3/1, Add5/1, Gain3/1
  Gain/1 -> Add2/1
  Unit Delay3/1 -> Product7/2, Unit Delay4/1
  Add2/1 -> Product7/1
  Gain1/1 -> Product8/1
  Product8/1 -> Add3/2, Add5/2
  Unit Delay4/1 -> Product9/2
  Add3/1 -> Product9/1
  Product9/1 -> Add4/2
  Product7/1 -> Add4/1
  Add4/1 -> Add1/2
  Add1/1 -> Divide/1
  Add5/1 -> Divide/2
  Gain2/1 -> Product2/2
  Gain3/1 -> Add2/2
  Product5/1 -> Product/1, Product/2, Product8/2
  const/1 -> Product5/1
  cutOff-Freq/1 -> Product5/2
  const3/1 -> Divide1/1
  samplingTime/1 -> Divide1/2
  Divide1/1 -> Gain1/1, Product4/2, Product4/1

== system CobiCalibration/Double-Click Button to set current folder ==

== stateflow chart CobiCalibration/getCalibrationAngle ==
  state init
    en:
    GCA_calibFlag = uint8(0);
    GCA_mountingSetup = int16(1);
    GCA_curMountingAngle_rad = single(0);
    GCA_mountingAngleFitlered_rad = single(0);
    GCA_firstEstimation = int16(1);
    GCA_minSpeed_kmh = single(7);
    GCA_calibrationFlag = uint8(0);
    GCA_reinitCounter = single(0);
  state getPreviousCalibInformation
    en:
    if GCA_initMountingSetup ~= 0 && abs(GCA_initMountingAngleRad) >=0.001
    %GCA_mountingSetup = GCA_initMountingSetup;
    GCA_mountingAngleFitlered_rad = GCA_initMountingAngleRad;
    GCA_calibrationFlag = uint8(1);
    GCA_firstEstimation = int16(0);
    end
  state idle
    en:
    GCA_lastSpeed_kmh = GCA_curSpeed_kmh;
    if GCA_calibrationFlag == 2
    GCA_calibrationFlag = uint8(1);
    end
  state ridingConstant
  state calibrating
    en:
    GCA_calibFlag = uint8(1);
    %detect mounting setup
    %if GCA_curAccSensorFrameFilteredX + sin(GCA_curSlope_rad) > 0  % 2 mounting possibilities with universal mount
    %    GCA_mountingSetup = int16(1);
    %else
    %    GCA_mountingSetup = int16(2);
    %end
    GCA_asinArg = GCA_curAccBikeFrameFilteredX/1000;
    if GCA_asinArg > 1  %saturation
    GCA_asinArg = single(1);
    elseif GCA_asinArg < -1
    GCA_asinArg = single(-1);
    end
    GCA_curMountingAngle_rad = asin(GCA_asinArg) + GCA_curSlope_rad; %this value represents the delta (not the overall) mounting angle
    if GCA_firstEstimation == 1
    GCA_mountingAngleFitlered_rad = -GCA_curMountingAngle_rad;
    GCA_firstEstimation = int16(0);
    %check reinitilization
    elseif abs(abs(GCA_mountingAngleFitlered_rad)-abs(GCA_curMountingAngle_rad)) >= 0.1 && ...
    abs(GCA_curMountingAngle_rad) >= 0.1
    GCA_reinitCounter = GCA_reinitCounter + 1;
    %do reinizialisation, no usage of low pass filtered mounting angle, new mounting angle is the current mounting angle estimation
    if GCA_reinitCounter >= 3
    GCA_asinArgSf = GCA_curAccSensorFrameFilteredX/1000;
    if GCA_asinArgSf > 1 %saturation
    GCA_asinArgSf = single(1);
    elseif GCA_asinArgSf < -1
    GCA_asinArgSf = single(-1);
    end
    GCA_mountingAngleFitlered_rad= asin(GCA_asinArgSf) + GCA_curSlope_rad;
    GCA_reinitCounter = single(0);
    GCA_calibrationFlag = uint8(2);
    else
    GCA_curMountingAngle_rad = asin(GCA_asinArg) + GCA_curSlope_rad;
    GCA_mountingAngleFitlered_rad = GCA_mountingAngleFitlered_rad - 1/10*GCA_curMountingAngle_rad;
    end
    else
    GCA_mountingAngleFitlered_rad = GCA_mountingAngleFitlered_rad - 1/10*GCA_curMountingAngle_rad;
    GCA_reinitCounter = single(0);
    end
    %if the currently estimated delta regarding the mounting angle is smaller 4.5°, the calibration flag is set to 1, this needs at least 2 mounting angle estimations!
    if abs(GCA_curMountingAngle_rad) < 0.08 && GCA_calibrationFlag ~= 2
    GCA_calibrationFlag = uint8(1);
    end
  (default) -> init
  init -> getPreviousCalibInformation : [after(3,sec)]
  getPreviousCalibInformation -> idle
  idle -> ridingConstant : [GCA_curSpeed_kmh >= GCA_minSpeed_kmh && ...
      | abs(GCA_curGyrBfFilteredY) <= 10000 && ...
      | abs(GCA_curSlope_rad) < 0.35 ...% no calibration if the extimated slope is greater +-20°
      | ]
  ridingConstant -> calibrating [order 2] : [after(3,sec)]
  ridingConstant -> idle [order 1] : [abs(GCA_curSpeed_kmh - GCA_lastSpeed_kmh) > 2 ... %1.5
      | || GCA_curSpeed_kmh < GCA_minSpeed_kmh || ...
      | abs(GCA_curAccBfFilteredY) > 250 || ...
      | abs(GCA_curGyrBfFilteredY) > 10000 || ...
      | GCA_crashScenario >= 1 || ...
      | abs(GCA_curSlope_rad) >= 0.35 ...% no calibration if the extimated slope is greater +-20°
      | ]
  calibrating -> idle : [after(1,sec)]
      | {
      | GCA_calibFlag = uint8(0);
      | }
  data: GCA_curAccBikeFrameFilteredX input; GCA_curAccSensorFrameFilteredX input; GCA_curSpeed_kmh input; GCA_curSlope_rad input; GCA_calibFlag output; GCA_mountingSetup output; GCA_lastSpeed_kmh local; GCA_firstEstimation local; GCA_minSpeed_kmh local; GCA_mountingAngleFitlered_rad output; GCA_curMountingAngle_rad output; GCA_calibrationFlag output; GCA_curAccBfFilteredY input; GCA_reinitCounter output; GCA_curGyrBfFilteredY input; GCA_initMountingSetup input; GCA_initMountingAngleRad input; GCA_asinArg local; GCA_asinArgSf local; GCA_crashScenario input

== stateflow chart CobiCalibration/SlopeEstimation ==
  state NotRiding1 [parallel] [commented out]
    en:
  state Riding2 [parallel] [commented out]
    en:
    SE_initPressure = SE_curPressure;
    du:
    SE_deltaAltitude_m = 8434.7 * log(SE_curPressure/SE_initPressure);
    SE_slopePressureBased = atand(SE_deltaAltitude_m/(SE_curSpeed_kmh/3.6*SE_timeStep));
    SE_initPressure = SE_curPressure;
  state Slope1 [parallel]
    settings: executionOrder=1
    state NotRiding
      en:
      SE_2EstFlag = logical(0);
    state Riding
      en:
      SE_2EstFlag = logical(0);
      SE_initPressure = SE_curPressure;
      SE_curDistanceM = SE_curSpeed_kmh/3.6*SE_timeStep;
    state SpeedIntegration
      en:
      SE_curDistanceM = SE_curSpeed_kmh/3.6*SE_timeStep + SE_curDistanceM;
      SE_timer = SE_timeStep;
      du:
      SE_curDistanceM = SE_curSpeed_kmh/3.6*SE_timeStep + SE_curDistanceM;
      SE_timer = SE_timer + SE_timeStep;
      if SE_timer >= 1
      SE_2EstFlag = logical(1);
      end
    state Riding1
      en:
      SE_deltaAltitude_m = 8434.7 * log(SE_curPressure/SE_initPressure);
      SE_asinArg = SE_deltaAltitude_m/SE_curDistanceM;
      if SE_asinArg > 1
      SE_asinArg = single(1);
      elseif SE_asinArg <-1
      SE_asinArg = single(-1);
      end
      SE_slopePressureBased = asind(SE_asinArg);
    (default) -> Slope1.NotRiding : {SE_slopePressureBased = 0;}
    Slope1.SpeedIntegration -> Slope1.NotRiding [order 2] : [SE_curSpeed_kmh < 3]
    Slope1.Riding -> Slope1.NotRiding [order 1] : [SE_curSpeed_kmh < 3]
    Slope1.NotRiding -> Slope1.Riding : [SE_curSpeed_kmh >= 3]
    Slope1.Riding -> Slope1.SpeedIntegration [order 2]
    Slope1.SpeedIntegration -> Slope1.Riding1 [order 1] : [after(2,sec)]
    Slope1.Riding1 -> Slope1.Riding : {
        |
        | }
  state Slope2 [parallel]
    settings: executionOrder=2
    state NotRiding
      en:
    state Riding
      en:
      SE_initPressure2 = SE_curPressure;
      SE_curDistance2M = SE_curSpeed_kmh/3.6*SE_timeStep;
      SE_2EstFlag = logical(0);
    state Riding1
      en:
      SE_deltaAltitude_m = 8434.7 * log(SE_curPressure/SE_initPressure2);
      SE_asinArg = SE_deltaAltitude_m/SE_curDistance2M;
      if SE_asinArg > 1
      SE_asinArg = single(1);
      elseif SE_asinArg <-1
      SE_asinArg = single(-1);
      end
      SE_slopePressureBased = asind(SE_asinArg);
    state SpeedIntegration
      en:
      SE_curDistance2M = SE_curSpeed_kmh/3.6*SE_timeStep + SE_curDistance2M;
      du:
      SE_curDistance2M = SE_curSpeed_kmh/3.6*SE_timeStep + SE_curDistance2M;
    (default) -> Slope2.NotRiding : {
        | SE_slopePressureBased = single(0);
        | SE_2EstFlag = logical(0);
        | }
    Slope2.Riding1 -> Slope2.NotRiding
    Slope2.SpeedIntegration -> Slope2.NotRiding [order 2] : [SE_curSpeed_kmh < 3]
    Slope2.Riding -> Slope2.NotRiding [order 1] : [SE_curSpeed_kmh < 3]
    Slope2.NotRiding -> Slope2.Riding : [SE_curSpeed_kmh >= 3 && ...
        | SE_2EstFlag == true]
    Slope2.Riding -> Slope2.SpeedIntegration [order 2]
    Slope2.SpeedIntegration -> Slope2.Riding1 [order 1] : [after(2,sec)]
  (default) -> NotRiding1 [commented out] : {SE_slopePressureBased = 0;}
  Riding2 -> NotRiding1 [commented out] : [SE_curSpeed_kmh < 3]
  NotRiding1 -> Riding2 [commented out] : [SE_curSpeed_kmh >= 3]
  data: SE_curPressure input; SE_curSpeed_kmh input; SE_timeStep input; SE_slopePressureBased output; SE_initPressure local; SE_deltaAltitude_m local; SE_curDistanceM local; SE_curDistance2M local; SE_initPressure2 local; SE_timer output; SE_2EstFlag output; SE_asinArg local

== matlab function CobiCalibration/MATLAB Function ==
  data: installAngle_rad input; accBfX_mg output; accSfX_mg input; accSfY_mg input; accSfZ_mg input; gyrSfX_mdegs input; gyrSfY_mdegs input; gyrSfZ_mdegs input; accBfY_mg output; accBfZ_mg output; gyrBfX_mdegs output; gyrBfY_mdegs output; gyrBfZ_mdegs output; mountingSetup input
function [accBfX_mg, accBfY_mg, accBfZ_mg, gyrBfX_mdegs, ...
    gyrBfY_mdegs, gyrBfZ_mdegs] = rotateFcn(installAngle_rad, ...
    accSfX_mg, accSfY_mg, accSfZ_mg, gyrSfX_mdegs, ...
    gyrSfY_mdegs, gyrSfZ_mdegs, mountingSetup)

    %Rotation setup: smartphone mounting setup 1 -> home button right
    if mountingSetup == 1
        rotMat = single([cos(installAngle_rad) 0 -1*sin(installAngle_rad);...
            0 1 0;...
            sin(installAngle_rad) 0 cos(installAngle_rad);]);
    %Rotation setup: smartphone mounting setup 2 -> home button left     
    elseif mountingSetup == 2
        rotMat = single([-1*cos(-installAngle_rad) 0 -1*sin(-installAngle_rad);...
            0 -1 0;...
            -1*sin(-installAngle_rad) 0 cos(-installAngle_rad);]);
    else
        rotMat = single(eye(3,3));
    end
    
    
    %accBf_mg = single(rotMat * [accSfX_mg; accSfY_mg; accSfZ_mg]);
    %gyrBf_mdegs = single(rotMat * [gyrSfX_mdegs; gyrSfY_mdegs; gyrSfZ_mdegs]);
    rotMatRound = single(int32(rotMat*1e+06))/1e+06;
    accBf_mg = single(rotMatRound * [accSfX_mg; accSfY_mg; accSfZ_mg]);
    gyrBf_mdegs = single(rotMatRound * [gyrSfX_mdegs; gyrSfY_mdegs; gyrSfZ_mdegs]);
    
%     if gyrSfX_mdegs == 1586 && gyrSfY_mdegs == -3662 
%         fprintf('stop');
%     end
    
    accBfX_mg = accBf_mg(1);
    accBfY_mg = accBf_mg(2);
    accBfZ_mg = accBf_mg(3);
    gyrBfX_mdegs = gyrBf_mdegs(1);
    gyrBfY_mdegs = gyrBf_mdegs(2);
    gyrBfZ_mdegs = gyrBf_mdegs(3);
end
